simulink model "observer_minimo"  (R2015a)
settings: Solver=ode3  StartTime=0.0  StopTime=10.0  FixedStep=1e-6  RelTol=1e-3
values from neighbouring files (symbols this model uses):
  a = [0 1;0 0]    [ejemplo_jury.m]    (also in observer_minimum.m = [0 1;0 -1]; realim_state_pd.m = [0 1;0 -1])
  Aaux = Abb-Ko*Aab    [observer_minimum.m]    (also in realim_state_pd.m = cat(2, cat(1,a,-c),zeros(3,1)))
  b = [0;1]    [ejemplo_jury.m]    (also in observer_minimum.m = [0; 10]; realim_state_pd.m = [0; 10])
  Baux = Aaux*Ko+Aba+Ko*Aaa    [observer_minimum.m]    (also in realim_state_pd.m = cat(1,b,-d))
  c = [1 0]    [ejemplo_jury.m]    (also in observer_minimum.m; realim_state_pd.m)
  d = 0    [ejemplo_jury.m]    (also in observer_minimum.m; realim_state_pd.m)
  F = Bb-Ko*Ba    [observer_minimum.m]
  k1 = 2.39    [ejemplo_jury.m]    (also in observer_minimum.m = [8.8 2.3]; realim_state_pd.m = [8.8 2.3])
  k2 = 16    [observer_minimum.m]    (also in realim_state_pd.m)
  Ko = place(Abb',Aab',polos)'    [observer_minimum.m]    (also in realim_state_pd.m = [199; 9801])
settings Model: Creator=Jose Roldan  LastModifiedBy=Jose Roldan

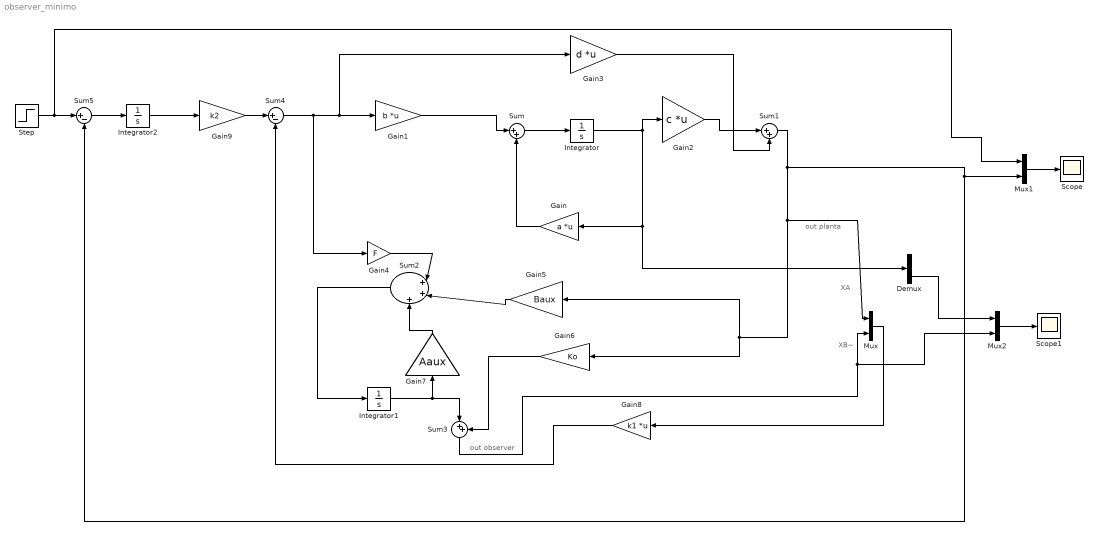
== system observer_minimo ==
  note: out planta
  note: out observer
  note: XB~
  note: XA
  Demux : Demux  Outputs=2
  Gain : Gain  Gain=a  Multiplication=Matrix(K*u)
  Gain1 : Gain  Gain=b  Multiplication=Matrix(K*u)
  Gain2 : Gain  Gain=c  Multiplication=Matrix(K*u)
  Gain3 : Gain  Gain=d  Multiplication=Matrix(K*u)
  Gain4 : Gain  Gain=F
  Gain5 : Gain  Gain=Baux
  Gain6 : Gain  Gain=Ko
  Gain7 : Gain  Gain=Aaux
  Gain8 : Gain  Gain=k1  Multiplication=Matrix(K*u)
  Gain9 : Gain  Gain=k2
  Integrator : Integrator
  Integrator1 : Integrator
  Integrator2 : Integrator
  Mux : Mux  Inputs=2
  Mux1 : Mux  Inputs=2
  Mux2 : Mux  Inputs=2
  Scope : Scope
      settings: YMin=0.999995  YMax=1.00007
  Scope1 : Scope
      settings: YMin=0  YMax=1.3
  Step : Step  SampleTime=0
  Sum : Sum  Inputs=|++
  Sum1 : Sum  Inputs=|++
  Sum2 : Sum  Inputs=|+++
  Sum3 : Sum  Inputs=|++
  Sum4 : Sum  Inputs=|+-
  Sum5 : Sum  Inputs=|+-
  wires:
  Gain1/1 -> Sum/1
  Sum/1 -> Integrator/1
  Integrator/1 -> Demux/1, Gain/1, Gain2/1
  Gain2/1 -> Sum1/1
  Gain3/1 -> Sum1/2
  Gain/1 -> Sum/2
  Gain4/1 -> Sum2/1
  Sum2/1 -> Integrator1/1
  Gain7/1 -> Sum2/3
  Integrator1/1 -> Sum3/1, Gain7/1
  Gain6/1 -> Sum3/2
  Sum1/1 -> Gain6/1, Gain5/1, Mux/1, Mux1/2, Sum5/2
  Gain5/1 -> Sum2/2
  Sum3/1 -> Mux2/2, Mux/2
  Mux/1 -> Gain8/1
  Gain8/1 -> Sum4/2
  Sum4/1 -> Gain4/1, Gain3/1, Gain1/1
  Sum5/1 -> Integrator2/1
  Integrator2/1 -> Gain9/1
  Gain9/1 -> Sum4/1
  Step/1 -> Mux1/1, Sum5/1
  Mux1/1 -> Scope/1
  Demux/2 -> Mux2/1
  Mux2/1 -> Scope1/1
